simulink model "simplified_suspension_model"  (R2020a)
settings: Solver=ode45  StartTime=0.0  StopTime=50  RelTol=1e-3
PreLoadFcn:
  | data_file
values from neighbouring files (symbols this model uses):
  current = 0.1:0.1:0.7    [data_file.m]
  d_force = [206.38 303.20 371.95 418.33 448.02 466.67 480.06]    [data_file.m]
undefined symbols (not defined in the file or in its folder): sigbuilder_block
settings Model: Creator=Viraj  LastModifiedBy=Viraj

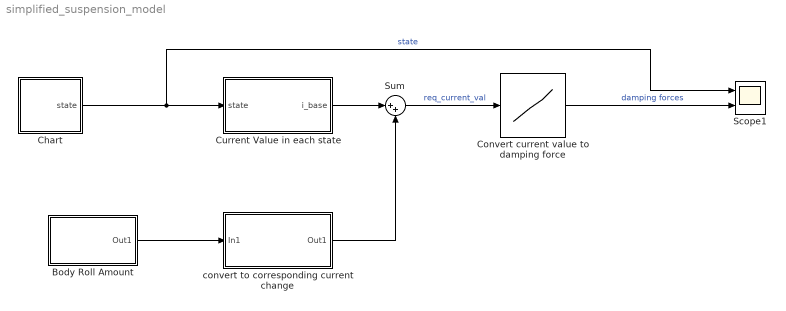
== system simplified_suspension_model ==
  Body Roll Amount : Subsystem
  Chart : Stateflow chart  TreatAsAtomicUnit=on
  Convert current value to damping force : Lookup_n-D  NumberOfTableDimensions=1  BreakpointsForDimension1=current  Table=d_force  InternalRulePriority=Speed  RndMeth=Simplest  InputSameDT=on
  Current Value in each state : MATLAB Function  TreatAsAtomicUnit=on
  Scope1 : Scope  NumInputPorts=2
  Sum : Sum  Inputs=|++
  convert to corresponding current change : Subsystem
  wires:
  Current Value in each state/1(i_base) -> Sum/1
  Chart/1(state) -> Scope1/1, Current Value in each state/1(state)  "state"
  Body Roll Amount/1(Out1) -> convert to corresponding current change/1(In1)
  Convert current value to damping force/1 -> Scope1/2  "damping forces"
  convert to corresponding current change/1(Out1) -> Sum/2
  Sum/1 -> Convert current value to damping force/1  "req_current_val"

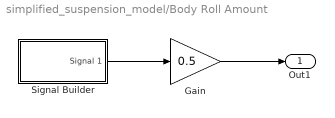
== system simplified_suspension_model/Body Roll Amount ==
  Gain : Gain  Gain=0.5
  Signal Builder : Subsystem  Tag=STV Subsys  LoadFcn=sigbuilder_block('load');  StartFcn=sigbuilder_block('start');  StopFcn=sigbuilder_block('stop');  ClipboardFcn=sigbuilder_block('clipboard');  mask(Sigbuilder block){tuvar=[0:10]}
      mask help: Simulink:masks:SigbuilderBlock_MD
      mask init:
      | if ~strcmp(get_param(bdroot(gcbh),'SimulationStatus'),'stopped') tuvar = sigbuilder_block('maskInit'); end
      settings: CopyFcn=sigbuilder_block('copy');  DeleteFcn=sigbuilder_block('delete');  ModelCloseFcn=sigbuilder_block('modelClose');  PreSaveFcn=sigbuilder_block('preSave');  PauseFcn=sigbuilder_block('pause');  ContinueFcn=sigbuilder_block('continue');  NameChangeFcn=sigbuilder_block('namechange');  OpenFcn=sigbuilder_block('open',[437.6 153 550.4 359.25 ]);  CloseFcn=sigbuilder_block('close');
      mask Display: plot(0, 0, 100, 100,[2, 2, 32, 32, 2], [68, 8, 8, 68, 68],[32, 2], [38, 38], [32, 19, 2],[53, 60, 44], [32, 17, 17, 2],[16, 16, 31, 31]);txt = getActiveGroup(gcbh);text(2, 100, txt,'verticalAlignment', 'top');
  Out1 : Outport
  wires:
  Signal Builder/1(Signal 1) -> Gain/1
  Gain/1 -> Out1/1

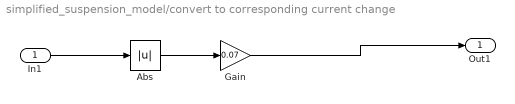
== system simplified_suspension_model/convert to corresponding current change ==
  In1 : Inport
  Abs : Abs
  Gain : Gain  Gain=0.07
  Out1 : Outport
  wires:
  In1/1 -> Abs/1
  Gain/1 -> Out1/1
  Abs/1 -> Gain/1

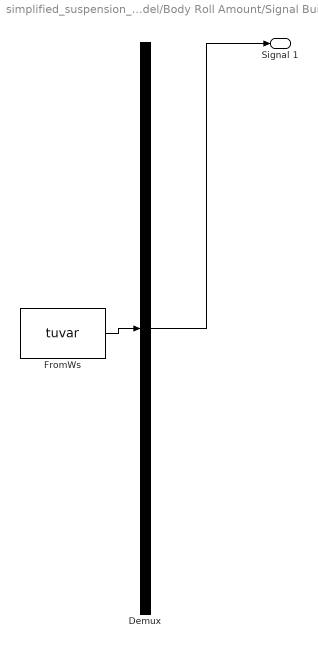
== system simplified_suspension_model/Body Roll Amount/Signal Builder ==
  Demux : Demux  Tag=STV Demux  Outputs=1
      settings: DisplayOption=none
  FromWs : FromWorkspace  Tag=STV FromWs  VariableName=tuvar
      SigBuilderData=|
      | common.afterFinalStr = 'Extrapolate'
      | common.sampleTime = 0
      | dataSet.timeRange = [0 50]
      | dataSet.name = 'Group 1'
      | sbobj.Groups.Name = 'Group 1'
      | sbobj.Groups.Signals.Name = 'Signal 1'
      | sbobj.Groups.Signals.XData = [0 0.1 0.2 0.3 0.4 0.5 0.6 0.7 0.8 0.9 1 1.1 ... (501 elements, 1x501)]
      | sbobj.Groups.Signals.YData = [0.109317693775 1.81401545028 0.312023828329 1.80449377172 -0.72312147957 0.52654703775 -0.260250861706 0.600142508809 0.593930795649 -2.18602161275 -1.32704314952 -1.44101359764 ... (501 elements, 1x501)]
      | sbobj.Groups.TimeRange = [0 50]
  Signal 1 : Outport  Tag=STV Outport
  wires:
  FromWs/1 -> Demux/1
  Demux/1 -> Signal 1/1

== matlab function simplified_suspension_model/Current Value in each state ==
  data: i_base output; state input
% This function is used to set the base current value in the MR damper
% solenoid

function i_base = fcn(state)

if (state == 0)
    i_base = 0.3;
elseif (state == 1)
    i_base = 0.5;
else
    i_base = 0.7;
end

end

== stateflow chart simplified_suspension_model/Chart ==
  state Comfort
    during:
    state = 0;
  state Sport
    during:
    state = 1;
  state Sport_plus
    during:
    state = 2;
  (default) -> Comfort
  Comfort -> Sport : after(15,sec)
  Sport_plus -> Comfort : after(15,sec)
  Sport -> Sport_plus : after(15,sec)
  data: state output
